simulink model "Control_path"  (R2021a)
settings: Solver=VariableStepAuto  StartTime=0.0  StopTime=90  RelTol=1e-3
undefined symbols (not defined in the file or in its folder): g, Ki, Kp, ksi, L, Te, vref, wref
libraries: simulink x17, pid_lib x2
settings Model: Creator=caios  LastModifiedBy=caios

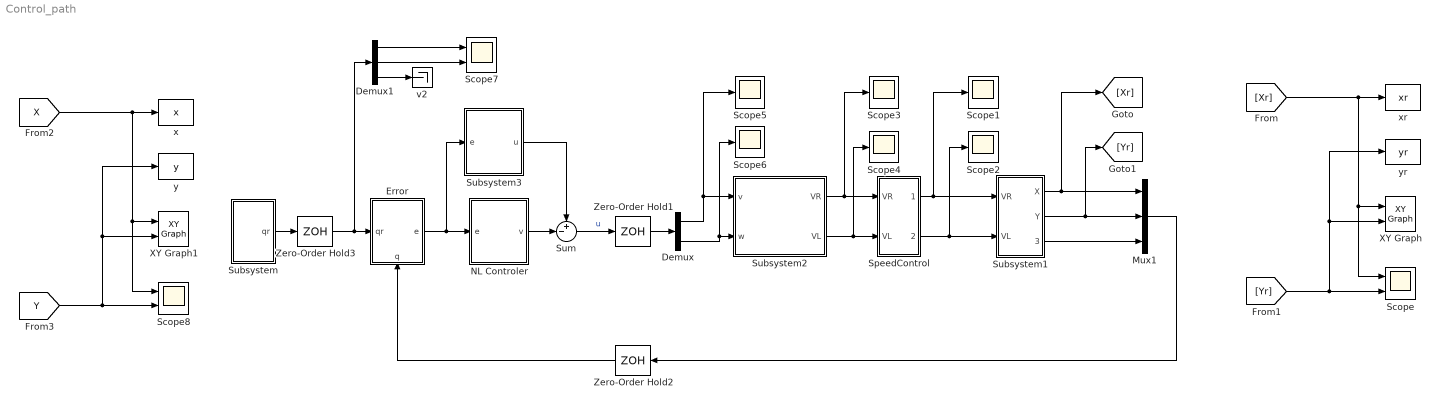
== system Control_path ==
  Demux : Demux  Outputs=2
  Demux1 : Demux  Outputs=3
  Error : Subsystem
      settings: PortSchema="{\"entries\":[{\"content\":{\"sides\":[{\"content\":{\"connectorIds\":[\"In1\"]},\"type\":\"ConnectorPlacement.EquallySpacedRectSide\",\"uuid\":\"a45b107d-ba29-4f75-869a-c56d8d13554a\"},{\"content\":{\"connectorIds\":[\"Out1\"],\"side\":\"RIGHT\"},\"type\":\"ConnectorPlacement.EquallySpacedRectSide\",\"uuid\":\"b5541495-130b-4cc3-b7e6-db691862bb12\"},{\"content\":{\"connectorIds\":[],\"side\":\"TOP\"},\"type\":\"ConnectorPlacement.EquallySpacedRectSide\",\"uuid\":\"8a05d011-71d6-4506-9719-787ac29c17b8\"},{\"content\":{\"connectorIds\":[\"In2\"],\"side\":\"BOTTOM\"},\"type\":\"ConnectorPlacement.EquallySpacedRectSide\",\"uuid\":\"9e355a0d-2c40-42a6-9622-b00ab7ea1076\"}]},\"type\":\"ConnectorPlacement.EquallySpacedConnector\",\"uuid\":\"e7bb514a-5c84-455e-8bdc-744a1a325939\"}],\"packageUris\":[\"http://schema.mathworks.com/mf0/Connector/R2020b\"],\"version\":\"1.0\"}"
  Mux1 : Mux  Inputs=3
  NL Controler : Subsystem
  Scope : Scope  NumInputPorts=2
  Scope{1..6} (6 alike) : Scope
  Scope7 : Scope  NumInputPorts=2
  Scope8 : Scope  NumInputPorts=2
  SpeedControl : Subsystem
  Subsystem : Subsystem
  Subsystem1 : Subsystem
  Subsystem2 : Subsystem
  Subsystem3 : Subsystem
  Sum : Sum  Inputs=+-|
  XY Graph : simulink/Sinks/XY Graph  xmin=0  xmax=3.3  ymin=0  ymax=3.3  st=-1
  XY Graph1 : simulink/Sinks/XY Graph  xmin=0  xmax=3.3  ymin=0  ymax=3.3  st=-1
  Zero-Order Hold1 : ZeroOrderHold  SampleTime=0.1
  Zero-Order Hold2 : ZeroOrderHold  SampleTime=0.1
  Zero-Order Hold3 : ZeroOrderHold  SampleTime=8
  v2 : Terminator
  x : ToWorkspace  VariableName=x  SaveFormat=Timeseries  SampleTime=-1
  xr : ToWorkspace  VariableName=xr  SaveFormat=Timeseries  SampleTime=-1
  y : ToWorkspace  VariableName=y  SaveFormat=Timeseries  SampleTime=-1
  yr : ToWorkspace  VariableName=yr  SaveFormat=Timeseries  SampleTime=-1
  wires:
  Subsystem1/1(X) -> Mux1/1, [Xr]
  Subsystem1/2(Y) -> Mux1/2, [Yr]
  Subsystem1/3(Theta) -> Mux1/3
  NL Controler/1(v) -> Sum/2
  Sum/1 -> Zero-Order Hold1/1  "u"
  Demux/1 -> Subsystem2/1(v), Scope5/1
  Demux/2 -> Scope6/1, Subsystem2/2(w)
  Subsystem3/1(u) -> Sum/1
  Mux1/1 -> Zero-Order Hold2/1
  Error/1(e) -> Subsystem3/1(e), NL Controler/1(e)
  SpeedControl/1(VRo) -> Subsystem1/1(VR), Scope1/1
  SpeedControl/2(VLo) -> Subsystem1/2(VL), Scope2/1
  Subsystem2/1(VR) -> SpeedControl/1(VR), Scope3/1
  Subsystem2/2(VL) -> SpeedControl/2(VL), Scope4/1
  Subsystem/1(qr) -> Zero-Order Hold3/1
  Zero-Order Hold1/1 -> Demux/1
  [Xr] -> Scope/1, XY Graph/1, xr/1
  [Yr] -> yr/1, XY Graph/2, Scope/2
  [X] -> Scope8/1, XY Graph1/1, x/1
  [Y] -> y/1, XY Graph1/2, Scope8/2
  Zero-Order Hold2/1 -> Error/2(q)
  Demux1/1 -> Scope7/1
  Demux1/2 -> Scope7/2
  Demux1/3 -> v2/1
  Zero-Order Hold3/1 -> Demux1/1, Error/1(qr)

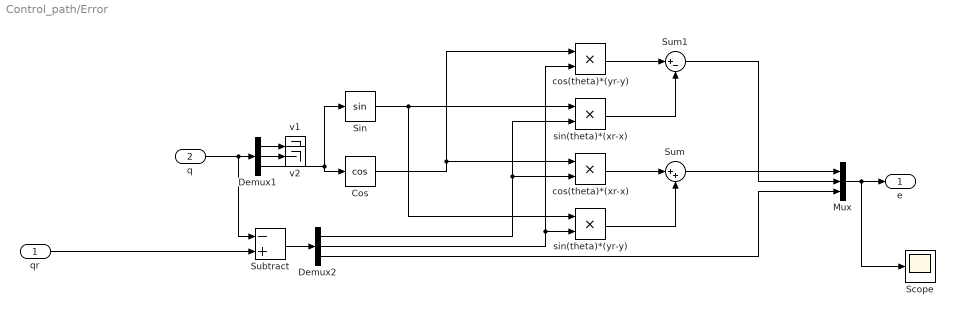
== system Control_path/Error ==
  qr : Inport
  q : Inport  Port=2
  Cos : Trigonometry  Operator=cos
  Demux1 : Demux  Outputs=3
  Demux2 : Demux  Outputs=3
  Mux : Mux  Inputs=3
  Scope : Scope
  Sin : Trigonometry
  Subtract : Sum  Inputs=-+
  Sum : Sum  Inputs=|++
  Sum1 : Sum  Inputs=|+-
  cos(theta)*(xr-x) : Product
  cos(theta)*(yr-y) : Product
  sin(theta)*(xr-x) : Product
  sin(theta)*(yr-y) : Product
  v1 : Terminator
  v2 : Terminator
  e : Outport
  wires:
  q/1 -> Demux1/1, Subtract/1
  Demux1/3 -> Sin/1, Cos/1
  Subtract/1 -> Demux2/1
  qr/1 -> Subtract/2
  Demux2/2 -> cos(theta)*(yr-y)/2, sin(theta)*(yr-y)/2
  Demux2/1 -> sin(theta)*(xr-x)/2, cos(theta)*(xr-x)/2
  Cos/1 -> cos(theta)*(yr-y)/1, cos(theta)*(xr-x)/1
  Sin/1 -> sin(theta)*(yr-y)/1, sin(theta)*(xr-x)/1
  cos(theta)*(xr-x)/1 -> Sum/1
  sin(theta)*(yr-y)/1 -> Sum/2
  sin(theta)*(xr-x)/1 -> Sum1/2
  cos(theta)*(yr-y)/1 -> Sum1/1
  Sum/1 -> Mux/1
  Sum1/1 -> Mux/2
  Demux1/1 -> v1/1
  Demux1/2 -> v2/1
  Demux2/3 -> Mux/3
  Mux/1 -> Scope/1, e/1

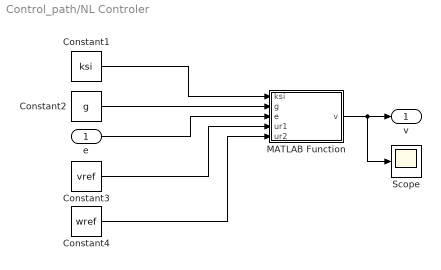
== system Control_path/NL Controler ==
  e : Inport
  Constant1 : Constant  Value=ksi
  Constant2 : Constant  Value=g
  Constant3 : Constant  Value=vref
  Constant4 : Constant  Value=wref
  MATLAB Function : MATLAB Function  TreatAsAtomicUnit=on
  Scope : Scope
  v : Outport
  wires:
  e/1 -> MATLAB Function/3(e)
  Constant1/1 -> MATLAB Function/1(ksi)
  Constant2/1 -> MATLAB Function/2(g)
  MATLAB Function/1(v) -> Scope/1, v/1
  Constant3/1 -> MATLAB Function/4(ur1)
  Constant4/1 -> MATLAB Function/5(ur2)

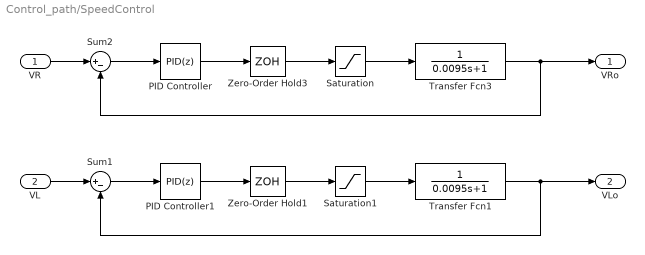
== system Control_path/SpeedControl ==
  VR : Inport
  VL : Inport  Port=2
  PID Controller : pid_lib/PID Controller  Controller=PID  Form=Parallel  TimeDomain=Discrete-time  UseExternalTs=off  SampleTime=Te  IntegratorMethod=Forward Euler  FilterMethod=Forward Euler  ControllerParametersSource=internal  P=Kp  I=Ki  D=0  UseFilter=off  N=100  TunerSelectOption=Transfer Function Based (PID Tuner App)  InitialConditionSource=internal  InitialConditionForIntegrator=0  InitialConditionForFilter=0  DifferentiatorICPrevScaledInput=0  ExternalReset=none  TrackingMode=off  Kt=1  LimitOutput=off  SatLimitsSource=internal  UpperSaturationLimit=inf  LowerSaturationLimit=-inf  LinearizeAsGain=on  AntiWindupMode=none  Kb=1  POutMin=[]  POutMax=[]  IOutMin=[]  IOutMax=[]  DOutMin=[]  DOutMax=[]  NOutMin=[]  NOutMax=[]  SumOutMin=[]  SumOutMax=[]  SaturationOutMin=[]  SaturationOutMax=[]  PParamMin=[]  PParamMax=[]  IParamMin=[]  IParamMax=[]  DParamMin=[]  DParamMax=[]  NParamMin=[]  NParamMax=[]  KbParamMin=[]  KbParamMax=[]  KtParamMin=[]  KtParamMax=[]  KbOutMin=[]  KbOutMax=[]  KtOutMin=[]  KtOutMax=[]  IntegratorOutMin=[]  IntegratorOutMax=[]  FilterOutMin=[]  FilterOutMax=[]  SumI1OutMin=[]  SumI1OutMax=[]  SumI2OutMin=[]  SumI2OutMax=[]  SumI3OutMin=[]  SumI3OutMax=[]  SumI4OutMin=[]  SumI4OutMax=[]  SumDOutMin=[]  SumDOutMax=[]  DifferentiatorOutMin=[]  DifferentiatorOutMax=[]  FilterDiffOutCoefMin=[]  FilterDiffOutCoefMax=[]  ReciprocalOutMin=[]  ReciprocalOutMax=[]  SumDenOutMin=[]  SumDenOutMax=[]  SumNumOutMin=[]  SumNumOutMax=[]  DivideOutMin=[]  DivideOutMax=[]  UdiffTsProdOutMin=[]  UdiffTsProdOutMax=[]  NTsProdOutMin=[]  NTsProdOutMax=[]  UintegralTsProdOutMin=[]  UintegralTsProdOutMax=[]  UngainTsProdOutMin=[]  UngainTsProdOutMax=[]  IntegratorContinuousStateAttributes=''  IntegratorStateMustResolveToSignalObject=off  IntegratorRTWStateStorageClass=Auto  FilterContinuousStateAttributes=''  FilterStateMustResolveToSignalObject=off  FilterRTWStateStorageClass=Auto  ParallelPVariant=InternalParameters  IdealPVariant=Disabled  IVariant=InternalParameters  DVariant=InternalParameters  IntegratorVariant=Discrete  SatVariant=Disabled  AWVariant=Passthrough  PCopyVariant=Disabled  TRVariant=Disabled  FdbkBlocksVariant=Forward  IdealPFdbkVariant=Disabled  SatFdbkVariant=Disabled  DerivativeFilterVariant=Differentiator  NVariant=Passthrough  NCopyVariant=Disabled_SignalSpec  FilterICVariant=InternalICsDifferentiator  IntegratorICVariant=InternalICs  ExternalResetVariant=Disabled  TRSumVariant=Passthrough  SumFdbkVariant=Disabled  SumVariant=Sum_PID  TsampFilterVariant=InternalTs  TsampNgainVariant=Passthrough  TsampIntegralVariant=Passthrough  ExternalSaturationOutDataTypeStr=Inherit: Same as second input
  PID Controller1 : pid_lib/PID Controller  Controller=PID  Form=Parallel  TimeDomain=Discrete-time  UseExternalTs=off  SampleTime=Te  IntegratorMethod=Forward Euler  FilterMethod=Forward Euler  ControllerParametersSource=internal  P=Kp  I=Ki  D=0  UseFilter=off  N=100  TunerSelectOption=Transfer Function Based (PID Tuner App)  InitialConditionSource=internal  InitialConditionForIntegrator=0  InitialConditionForFilter=0  DifferentiatorICPrevScaledInput=0  ExternalReset=none  TrackingMode=off  Kt=1  LimitOutput=off  SatLimitsSource=internal  UpperSaturationLimit=inf  LowerSaturationLimit=-inf  LinearizeAsGain=on  AntiWindupMode=none  Kb=1  POutMin=[]  POutMax=[]  IOutMin=[]  IOutMax=[]  DOutMin=[]  DOutMax=[]  NOutMin=[]  NOutMax=[]  SumOutMin=[]  SumOutMax=[]  SaturationOutMin=[]  SaturationOutMax=[]  PParamMin=[]  PParamMax=[]  IParamMin=[]  IParamMax=[]  DParamMin=[]  DParamMax=[]  NParamMin=[]  NParamMax=[]  KbParamMin=[]  KbParamMax=[]  KtParamMin=[]  KtParamMax=[]  KbOutMin=[]  KbOutMax=[]  KtOutMin=[]  KtOutMax=[]  IntegratorOutMin=[]  IntegratorOutMax=[]  FilterOutMin=[]  FilterOutMax=[]  SumI1OutMin=[]  SumI1OutMax=[]  SumI2OutMin=[]  SumI2OutMax=[]  SumI3OutMin=[]  SumI3OutMax=[]  SumI4OutMin=[]  SumI4OutMax=[]  SumDOutMin=[]  SumDOutMax=[]  DifferentiatorOutMin=[]  DifferentiatorOutMax=[]  FilterDiffOutCoefMin=[]  FilterDiffOutCoefMax=[]  ReciprocalOutMin=[]  ReciprocalOutMax=[]  SumDenOutMin=[]  SumDenOutMax=[]  SumNumOutMin=[]  SumNumOutMax=[]  DivideOutMin=[]  DivideOutMax=[]  UdiffTsProdOutMin=[]  UdiffTsProdOutMax=[]  NTsProdOutMin=[]  NTsProdOutMax=[]  UintegralTsProdOutMin=[]  UintegralTsProdOutMax=[]  UngainTsProdOutMin=[]  UngainTsProdOutMax=[]  IntegratorContinuousStateAttributes=''  IntegratorStateMustResolveToSignalObject=off  IntegratorRTWStateStorageClass=Auto  FilterContinuousStateAttributes=''  FilterStateMustResolveToSignalObject=off  FilterRTWStateStorageClass=Auto  ParallelPVariant=InternalParameters  IdealPVariant=Disabled  IVariant=InternalParameters  DVariant=InternalParameters  IntegratorVariant=Discrete  SatVariant=Disabled  AWVariant=Passthrough  PCopyVariant=Disabled  TRVariant=Disabled  FdbkBlocksVariant=Forward  IdealPFdbkVariant=Disabled  SatFdbkVariant=Disabled  DerivativeFilterVariant=Differentiator  NVariant=Passthrough  NCopyVariant=Disabled_SignalSpec  FilterICVariant=InternalICsDifferentiator  IntegratorICVariant=InternalICs  ExternalResetVariant=Disabled  TRSumVariant=Passthrough  SumFdbkVariant=Disabled  SumVariant=Sum_PID  TsampFilterVariant=InternalTs  TsampNgainVariant=Passthrough  TsampIntegralVariant=Passthrough  ExternalSaturationOutDataTypeStr=Inherit: Same as second input
  Saturation : Saturate  UpperLimit=0.274  LowerLimit=-0.15
  Saturation1 : Saturate  UpperLimit=0.274  LowerLimit=-0.15
  Sum1 : Sum  Inputs=|+-
  Sum2 : Sum  Inputs=|+-
  Transfer Fcn1 : TransferFcn  Denominator=[0.0095 1]
  Transfer Fcn3 : TransferFcn  Denominator=[0.0095 1]
  Zero-Order Hold1 : ZeroOrderHold  SampleTime=Te
  Zero-Order Hold3 : ZeroOrderHold  SampleTime=Te
  VRo : Outport
  VLo : Outport  Port=2
  wires:
  PID Controller/1 -> Zero-Order Hold3/1
  Transfer Fcn3/1 -> VRo/1, Sum2/2
  Zero-Order Hold3/1 -> Saturation/1
  Saturation/1 -> Transfer Fcn3/1
  Sum2/1 -> PID Controller/1
  VR/1 -> Sum2/1
  PID Controller1/1 -> Zero-Order Hold1/1
  VL/1 -> Sum1/1
  Transfer Fcn1/1 -> VLo/1, Sum1/2
  Sum1/1 -> PID Controller1/1
  Saturation1/1 -> Transfer Fcn1/1
  Zero-Order Hold1/1 -> Saturation1/1

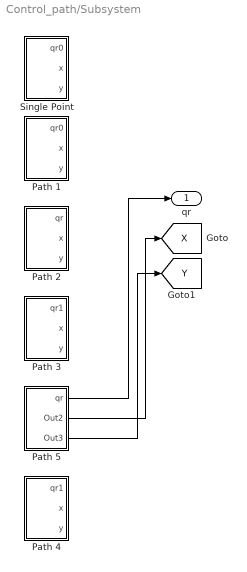
== system Control_path/Subsystem ==
  Path 1 : Subsystem
  Path 2 : Subsystem
  Path 3 : Subsystem
  Path 4 : Subsystem
  Path 5 : Subsystem
  Single Point : Subsystem
  qr : Outport
  tag scope: X=global, Y=global
  wires:
  Path 5/1(qr) -> qr/1
  Path 5/2(Out2) -> [X]
  Path 5/3(Out3) -> [Y]

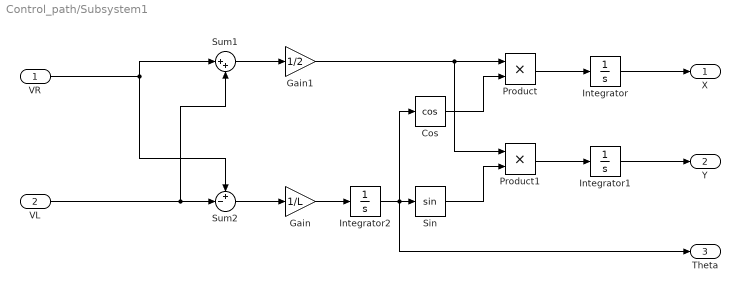
== system Control_path/Subsystem1 ==
  VR : Inport
  VL : Inport  Port=2
  Cos : Trigonometry  Operator=cos
  Gain : Gain  Gain=1/L
  Gain1 : Gain  Gain=1/2
  Integrator : Integrator
  Integrator1 : Integrator
  Integrator2 : Integrator
  Product : Product
  Product1 : Product
  Sin : Trigonometry
  Sum1 : Sum  Inputs=|++
  Sum2 : Sum  Inputs=+-|
  X : Outport
  Y : Outport  Port=2
  Theta : Outport  Port=3
  wires:
  Integrator/1 -> X/1
  Product/1 -> Integrator/1
  Integrator2/1 -> Cos/1, Sin/1, Theta/1
  Integrator1/1 -> Y/1
  Sin/1 -> Product1/2
  Product1/1 -> Integrator1/1
  Cos/1 -> Product/2
  Gain/1 -> Integrator2/1
  Gain1/1 -> Product1/1, Product/1
  VR/1 -> Sum2/1, Sum1/1
  Sum2/1 -> Gain/1
  VL/1 -> Sum2/2, Sum1/2
  Sum1/1 -> Gain1/1

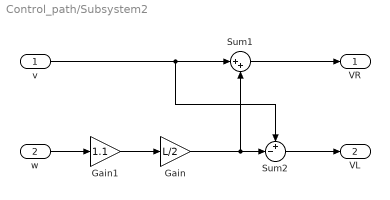
== system Control_path/Subsystem2 ==
  v : Inport
  w : Inport  Port=2
  Gain : Gain  Gain=L/2
  Gain1 : Gain  Gain=1.1
  Sum1 : Sum  Inputs=|++
  Sum2 : Sum  Inputs=+-|
  VR : Outport
  VL : Outport  Port=2
  wires:
  v/1 -> Sum1/1, Sum2/1
  Gain/1 -> Sum2/2, Sum1/2
  Sum1/1 -> VR/1
  Sum2/1 -> VL/1
  w/1 -> Gain1/1
  Gain1/1 -> Gain/1

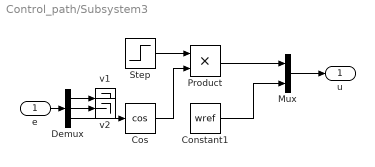
== system Control_path/Subsystem3 ==
  e : Inport
  Constant1 : Constant  Value=wref
  Cos : Trigonometry  Operator=cos
  Demux : Demux  Outputs=3
  Mux : Mux  Inputs=2
  Product : Product
  Step : Step  After=vref  SampleTime=0
  v1 : Terminator
  v2 : Terminator
  u : Outport
  wires:
  Demux/1 -> v1/1
  Demux/2 -> v2/1
  Mux/1 -> u/1
  Cos/1 -> Product/2
  Demux/3 -> Cos/1
  Product/1 -> Mux/1
  e/1 -> Demux/1
  Step/1 -> Product/1
  Constant1/1 -> Mux/2

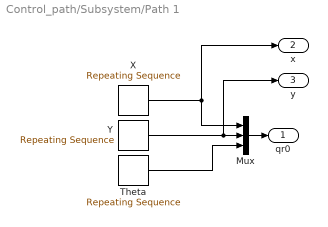
== system Control_path/Subsystem/Path 1 ==
  Mux : Mux  Inputs=3
  Theta : simulink/Sources/Repeating Sequence  rep_seq_t=10*[0 0.9999 1 1.9999 2 2.9999 3 3.9999 4 4.9999 5 10 100]  rep_seq_y=[0 0 0.785 0.785 1.57 1.57 2.355 2.355 3.14 3.14 3.14 3.14 3.14]
  X : simulink/Sources/Repeating Sequence  rep_seq_t=10*[0 1 2 3 4 5 10 100]  rep_seq_y=5*[0 0.1 0.171 0.171 0.1 0 0 0]
  Y : simulink/Sources/Repeating Sequence  rep_seq_t=10*[0 1 2 3 4 5 10 100]  rep_seq_y=5*[0 0 0.071 0.171 0.242 0.242 0.242 0.242]
  qr0 : Outport
  x : Outport  Port=2
  y : Outport  Port=3
  wires:
  X/1 -> Mux/1, x/1
  Y/1 -> y/1, Mux/2
  Theta/1 -> Mux/3
  Mux/1 -> qr0/1

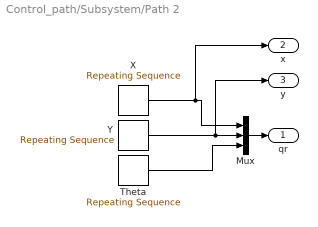
== system Control_path/Subsystem/Path 2 ==
  Mux : Mux  Inputs=3
  Theta : simulink/Sources/Repeating Sequence  rep_seq_t=5*[0 0.999 1 1.999 2 2.999 3 3.999 4 4.999 5 5.999 6 6.999 7 7.999 8 8.999 9 9.999 10 10.999 11 11.999 100]  rep_seq_y=[0 0 0 0 1.57 1.57 1.57 1.57 0 0 0 0 0 0 -1.57 -1.57 -1.57 -1.57 0 0 0 0 0 0 0]
  X : simulink/Sources/Repeating Sequence  rep_seq_t=5*[0 1 2 3 4 5 6 7 8 9 10 11 12 100]  rep_seq_y=2*[0 0.1 0.2 0.2 0.2 0.3 0.4 0.5 0.5 0.5 0.6 0.7 0.8 0.8]
  Y : simulink/Sources/Repeating Sequence  rep_seq_t=5*[0 1 2 3 4 5 6 7 8 9 10 11 12 100]  rep_seq_y=2*[0 0 0 0.1 0.2 0.2 0.2 0.2 0.1 0 0 0 0 0]
  qr : Outport
  x : Outport  Port=2
  y : Outport  Port=3
  wires:
  Theta/1 -> Mux/3
  Mux/1 -> qr/1
  Y/1 -> y/1, Mux/2
  X/1 -> x/1, Mux/1

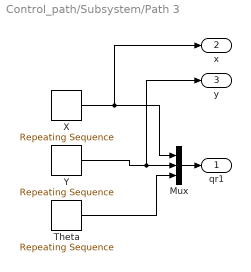
== system Control_path/Subsystem/Path 3 ==
  Mux : Mux  Inputs=3
  Theta : simulink/Sources/Repeating Sequence  rep_seq_t=[0 3.99999 4 7.99999 8 11.99999 12 15.99999 16 100]  rep_seq_y=[0 0 0 0 1.57 1.57 3.14 3.14 3.14 3.14]
  X : simulink/Sources/Repeating Sequence  rep_seq_t=[0 4 8 12 16 100]  rep_seq_y=[0 3 6 6 3 3]
  Y : simulink/Sources/Repeating Sequence  rep_seq_t=[0 4 8 12 16 100]  rep_seq_y=[0 3 3 6 6 6]
  qr1 : Outport
  x : Outport  Port=2
  y : Outport  Port=3
  wires:
  Theta/1 -> Mux/3
  Mux/1 -> qr1/1
  Y/1 -> y/1, Mux/2
  X/1 -> x/1, Mux/1

== system Control_path/Subsystem/Path 4 ==
  Mux : Mux  Inputs=3
  Theta : simulink/Sources/Repeating Sequence  rep_seq_t=5*[0 3.9999 4 7.99 8 11.9999 12 15.9999 16 17.9999 18 19.9999 20 100]  rep_seq_y=[0 0 0 0 1.57 1.57 1.57 1.57 3.14 3.14 3.14 3.14 3.14 3.14]
  X : simulink/Sources/Repeating Sequence  rep_seq_t=5*[0 4 8 12 16 18 20 100]  rep_seq_y=[0 0.75 1.5 1.5 1.5 0.75 0 0]
  Y : simulink/Sources/Repeating Sequence  rep_seq_t=5*[0 4 8 12 16 18 20 100]  rep_seq_y=[0 0 0 0.75 1.5 1.5 1.5 1.5]
  qr1 : Outport
  x : Outport  Port=2
  y : Outport  Port=3
  wires:
  Theta/1 -> Mux/3
  Mux/1 -> qr1/1
  Y/1 -> y/1, Mux/2
  X/1 -> x/1, Mux/1

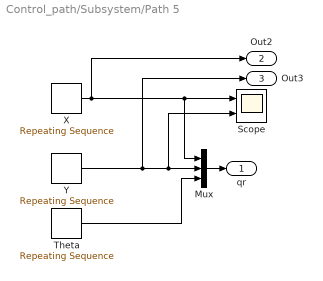
== system Control_path/Subsystem/Path 5 ==
  Mux : Mux  Inputs=3
  Scope : Scope  NumInputPorts=2
  Theta : simulink/Sources/Repeating Sequence  rep_seq_t=5*[0 3.99 4 7.99 8 11.99 12 15.99 16 100]  rep_seq_y="[0.78  0.78 0 0 1.57 1.57 3.14 3.14 3.14 3.14]"
  X : simulink/Sources/Repeating Sequence  rep_seq_t=5*[0 4 8 12 16 100]  rep_seq_y=0.25*[0 4 8 8 4 4]
  Y : simulink/Sources/Repeating Sequence  rep_seq_t=5*[0 4 8 12 16 100]  rep_seq_y=0.25*[0 4 4 8 8 8]
  qr : Outport
  Out2 : Outport  Port=2
  Out3 : Outport  Port=3
  wires:
  Theta/1 -> Mux/3
  Y/1 -> Out3/1, Scope/2, Mux/2
  Mux/1 -> qr/1
  X/1 -> Out2/1, Mux/1, Scope/1

== system Control_path/Subsystem/Single Point ==
  Mux : Mux  Inputs=3
  Step : Step  After=1.5  SampleTime=0
  Step1 : Step  After=1.5  SampleTime=0
  Step2 : Step  Time=0  After=1.57  SampleTime=0
  qr0 : Outport
  x : Outport  Port=2
  y : Outport  Port=3
  wires:
  Step/1 -> Mux/1, x/1
  Mux/1 -> qr0/1
  Step2/1 -> Mux/3
  Step1/1 -> y/1, Mux/2

== matlab function Control_path/NL Controler/MATLAB Function ==
  data: ksi input; v output; g input; e input; ur1 input; ur2 input
function v = fcn(ksi, g, e, ur1, ur2)

wn = sqrt(ur2^2+g*(ur1^2));

k1 = 2*ksi*wn;
k2 = g*abs(ur1);
k3 = k1;


K = [-k1       0          0;
      0  -sign(ur1)*k2   -k3 ];
  
  
  
v = K*e;
